simulink model "step2"  (R2023a)
settings: Solver=ode4  StartTime=0.0  StopTime=10.0  RelTol=1e-3
values from neighbouring files (symbols this model uses):
  K = 1    [nyquist.m]
settings Model: Creator=hi  LastModifiedBy=hi
settings DataIOCC: ReturnWorkspaceOutputs=off

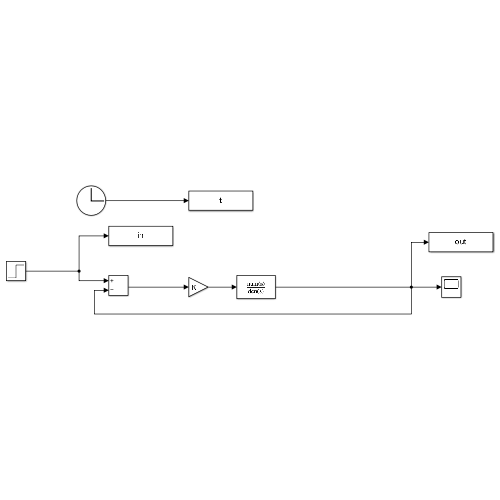
[thumbnail: Simulink's stored preview of the top-level diagram]
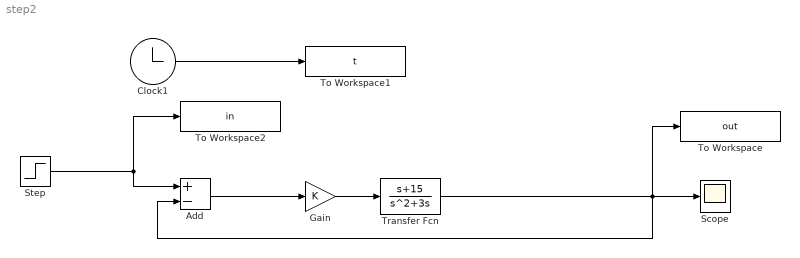
== system step2 ==
  Add : Sum  Inputs=+-
  Clock1 : Clock
  Gain : Gain  Gain=K
  Scope : Scope
  Step : Step  Time=0  OutDataTypeStr=Inherit: Inherit via back propagation  SampleTime=0
  To Workspace : ToWorkspace  VariableName=out  SampleTime=-1
  To Workspace1 : ToWorkspace  VariableName=t  SampleTime=-1
  To Workspace2 : ToWorkspace  VariableName=in  SampleTime=-1
  Transfer Fcn : TransferFcn  Numerator=[1 15]  Denominator=[1 3 0]
  wires:
  Clock1/1 -> To Workspace1/1
  Step/1 -> Add/1, To Workspace2/1
  Gain/1 -> Transfer Fcn/1
  Add/1 -> Gain/1
  Transfer Fcn/1 -> Add/2, To Workspace/1, Scope/1
